simulink model "trajectory_gen"  (R2020b)
settings: Solver=VariableStepAuto  StartTime=0.0  StopTime=400  RelTol=1e-3
settings Model: Creator=shanerutherford  LastModifiedBy=shanerutherford

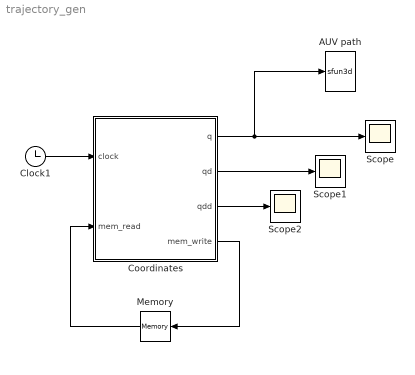
== system trajectory_gen ==
  AUV path : S-Function  LoadFcn=if exist('sfun3d','file'), sfun3d([],[],[],'LoadBlock'); end  FunctionName=sfun3d  Parameters=ax,T,np,cp,gd,ls,mk,mx,hd,tb  SFunctionDeploymentMode=off  EnableBusSupport=off  mask(3D Graph){np=1, ax=[-15 15 -15 15 -20 20], mx=1e4, T=-1, cp=[0, 0 15], gd=on, hd=on, tb=on, ls=-, mk=none}
      mask prompts: np "Number of moving points (lines)"; ax "Range: [xmin xmax  ymin ymax zmin zmax]"; mx "Max number of points in each line"; T "Sampling Time"; cp "Camera position (use [0 0 1] for 2D XY view)"; gd "Grid (on|off)"; hd "HeadMarkers (on|off)"; tb "Toolbar (on|off)"; ls "LineStyle"; mk "LineMarker"
      mask help:
      | This block plots the position of several points in the XYZ space. The input contains the coordinates of all the points (x1,y1,z1,x2,y2,z2,...).
      | The number of moving points (lines), the XYZ ranges, sampling time, camera position, and grid (among other things) can be set as mask parameters.
      settings: CopyFcn=if exist('sfun3d','file'), sfun3d([],[],[],'CopyBlock'); end  DeleteFcn=if exist('sfun3d','file'), sfun3d([],[],[],'DeleteBlock'); end  NameChangeFcn=if exist('sfun3d','file'), sfun3d([],[],[],'NameChange'); end
      mask Help:
      | This block plots the position of several points in the XYZ space. The input contains the coordinates of all the points (x1,y1,z1,x2,y2,z2,...).
      | The number of moving points (lines), the XYZ ranges, sampling time, camera position, and grid (among other things) can be set as mask parameters.
      mask TypeOptions ls: - | -- | : | -. | none
      mask TypeOptions mk: none | . | + | o | * | x | square | diamond | v | ^ | > | < | pentagram | hexagram
      mask Display: plot([.05 .95 .95 .05 .05],[.45 .45 .95 .95 .45], 0.5+cos(0:0.1:2*pi)*0.3,0.7+sin(0:0.1:2*pi)*0.2)
  Clock1 : Clock
  Coordinates : MATLAB Function  TreatAsAtomicUnit=on
  Memory : Memory  InitialCondition=zeros(7, 7)
  Scope : Scope
  Scope1 : Scope
  Scope2 : Scope
  wires:
  Coordinates/3(qdd) -> Scope2/1
  Coordinates/1(q) -> AUV path/1, Scope/1
  Coordinates/2(qd) -> Scope1/1
  Clock1/1 -> Coordinates/1(clock)
  Coordinates/4(mem_write) -> Memory/1
  Memory/1 -> Coordinates/2(mem_read)

== matlab function trajectory_gen/Coordinates ==
  data: q output; qd output; qdd output; clock input; mem_read input; mem_write output
function [q, qd, qdd, mem_write] = fcn(clock, mem_read)

    avg_speed = 0.8; % m/s
    
    
    % Should run one time to initalise waypoints
    if mem_read == 0
        wayPoints = [
            0, 10,   0, -10, 10,   0, -10;
            0, 10, -10,  10, 10, -10,  10;
            0,  0,   0,   0,  4,   4,   4; 
        ];
        timePoints = ones(1, 7);
        timePoints(1, 1) = 0;
        velocityPoints = zeros(3, 7);
    else
        wayPoints = mem_read(1:3, 1:7);
        timePoints = mem_read(4, 1:7);
        velocityPoints = mem_read(5:7, 1:7);
    end
    
    
    % generate a new random waypoint and rotate waypoints
    [~, n] = size(wayPoints);
    if clock > timePoints(1, 3)
        for i = 2:n
            wayPoints(1:3, i-1) = wayPoints(1:3, i);
            timePoints(1, i-1) = timePoints(1, i);
            velocityPoints(1:3, i-1) = velocityPoints(1:3, i);
        end
        wayPoints(1:3, n) = 20 * ([rand(1)-0.5; rand(1)-0.5; rand(1)-0.2]);
    end

    
    % Generate timepoints and velocity points
    for i = 2:n
        distance = norm(wayPoints(1:3, i) - wayPoints(1:3, i-1));
        timePoints(1, i) = timePoints(1, i-1) + distance/avg_speed;
    end
    
    for i = 2:n-1
        vector = wayPoints(1:3, i+1) - wayPoints(1:3, i-1);
        if abs(sum(vector)) < 0.1
            w = wayPoints(1:3, i) - wayPoints(1:3, i-1);
            vector = [-w(2); w(1); 0];
        end
        unit_d = vector / norm(vector);
        velocityPoints(1:3, i) = avg_speed*unit_d;
    end
    
    
    % Generate trajectory
    tSamples = timePoints(1, 1):0.001:timePoints(1, n);
    [Q, QD, QDD, ~] = cubicpolytraj(wayPoints, timePoints, tSamples, 'VelocityBoundaryCondition', velocityPoints);
    time_index = 1;
    [~, max_index] = size(tSamples);
    while tSamples(time_index) < clock
        time_index = time_index + 1;
        if time_index > max_index
            time_index = max_index;
            break
        end
    end
    q = Q(1:3, time_index);
    qd = QD(1:3, time_index);
    qdd = QDD(1:3, time_index);
    mem_write = [
        wayPoints; 
        timePoints;
        velocityPoints];
end
